simulink model "P702_NI_SoftECU"  (R2019a)
settings: Solver=ode1  StartTime=0.0  StopTime=Inf  FixedStep=0.001  RelTol=1e-3  EnableMultiTasking=on
PreLoadFcn:
  | run '.\VeriStand_BlockSet\NIVeriStandAddPaths.m'
undefined symbols (not defined in the file or in its folder): magnitude
libraries: simulink x83, simulink_extras x1
(part 63 of 76)

== system P702_NI_SoftECU/SoftECU/SCCM/Mapping/Steering_Data ==
  In1 : Inport
  Bus Selector : BusSelector  OutputSignals=AhbStat_B_Dsply,HeadLghtHiCtrl_D_RqAhb,HeadLghtHiOn_B_StatAhb,CcButtnOnPress,CcButtnOffPress,CcAslButtnCnclPress,CcAsllButtnResPress,CcAslButtnResIncPress,CcAslButtnSetIncPress,CcAslButtnSetDecPress,CcAslButtnSetPress,AccButtnGapIncPress,AccButtnGapDecPress,AslButtnOnOffPress,AslButtnOnOffCnclPress,CcButtnOnOffPress,CcButtnOnOffCnclPress,CcAslButtnResDecPress,CcAslButtnOnPress,CcAslButtnCnclResPress
  Gain{,1..19} (20 alike) : Gain
  buscreator : BusCreator  Inputs=20
  Out1 : Outport
  wires:
  buscreator/1 -> Out1/1  "Steering_Data"
  Bus Selector/1 -> Gain19/1  "<AhbStat_B_Dsply>"
  Bus Selector/2 -> Gain18/1  "<HeadLghtHiCtrl_D_RqAhb>"
  Bus Selector/3 -> Gain17/1  "<HeadLghtHiOn_B_StatAhb>"
  In1/1 -> Bus Selector/1
  Gain19/1 -> buscreator/1  "AhbStat_B_Dsply"
  Gain18/1 -> buscreator/2  "HeadLghtHiCtrl_D_RqAhb"
  Gain17/1 -> buscreator/3  "HeadLghtHiOn_B_StatAhb"
  Bus Selector/7 -> Gain13/1  "<CcAsllButtnResPress>"
  Bus Selector/5 -> Gain15/1  "<CcButtnOffPress>"
  Bus Selector/6 -> Gain14/1  "<CcAslButtnCnclPress>"
  Bus Selector/4 -> Gain16/1  "<CcButtnOnPress>"
  Bus Selector/8 -> Gain/1  "<CcAslButtnResIncPress>"
  Bus Selector/9 -> Gain1/1  "<CcAslButtnSetIncPress>"
  Bus Selector/10 -> Gain2/1  "<CcAslButtnSetDecPress>"
  Gain15/1 -> buscreator/5  "CcButtnOffPress"
  Gain1/1 -> buscreator/9  "CcAslButtnSetIncPress"
  Gain14/1 -> buscreator/6  "CcAslButtnCnclPress"
  Gain/1 -> buscreator/8  "CcAslButtnResIncPress"
  Gain13/1 -> buscreator/7  "CcAsllButtnResPress"
  Gain16/1 -> buscreator/4  "CcButtnOnPress"
  Gain2/1 -> buscreator/10  "CcAslButtnSetDecPress"
  Bus Selector/11 -> Gain3/1  "<CcAslButtnSetPress>"
  Gain3/1 -> buscreator/11  "CcAslButtnSetPress"
  Bus Selector/17 -> Gain9/1  "<CcButtnOnOffCnclPress>"
  Bus Selector/19 -> Gain11/1  "<CcAslButtnOnPress>"
  Bus Selector/15 -> Gain7/1  "<AslButtnOnOffCnclPress>"
  Bus Selector/16 -> Gain8/1  "<CcButtnOnOffPress>"
  Bus Selector/13 -> Gain5/1  "<AccButtnGapDecPress>"
  Bus Selector/20 -> Gain12/1  "<CcAslButtnCnclResPress>"
  Bus Selector/12 -> Gain4/1  "<AccButtnGapIncPress>"
  Bus Selector/14 -> Gain6/1  "<AslButtnOnOffPress>"
  Bus Selector/18 -> Gain10/1  "<CcAslButtnResDecPress>"
  Gain6/1 -> buscreator/14  "AslButtnOnOffPress"
  Gain7/1 -> buscreator/15  "AslButtnOnOffCnclPress"
  Gain5/1 -> buscreator/13  "AccButtnGapDecPress"
  Gain4/1 -> buscreator/12  "AccButtnGapIncPress"
  Gain11/1 -> buscreator/19  "CcAslButtnOnPress"
  Gain9/1 -> buscreator/17  "CcButtnOnOffCnclPress"
  Gain8/1 -> buscreator/16  "CcButtnOnOffPress"
  Gain12/1 -> buscreator/20  "CcAslButtnCnclResPress"
  Gain10/1 -> buscreator/18  "CcAslButtnResDecPress"

== system P702_NI_SoftECU/SoftECU/SCCM/Mapping/Steering_Wheel_Data2 ==
  In1 : Inport
  Bus Creator6 : BusCreator  Inputs=7
  Bus Selector : BusSelector  OutputSignals=SteWhlSwtchOk_B_Stat,SteeringWheelTglBtnUp_B,SteeringWheelTglBtnDown_B,SteeringWheelTglBtnLeft_B,SteeringWheelTglBtnRight_B,SteeringWheelTglBtnMenue_B,SteeringWheelTglBtnBack_B
  Gain{,1..6} (7 alike) : Gain
  Out1 : Outport
  wires:
  Bus Creator6/1 -> Out1/1  "Steering_Wheel_Data2"
  Gain/1 -> Bus Creator6/1  "SteWhlSwtchOk_B_Stat"
  Gain1/1 -> Bus Creator6/2  "SteWhlSwtchUp_B_Stat"
  Gain2/1 -> Bus Creator6/3  "SteWhlSwtchDown_B_Stat"
  Gain3/1 -> Bus Creator6/4  "SteWhlSwtchLeft_B_Stat"
  Gain4/1 -> Bus Creator6/5  "SteWhlSwtchRght_B_Stat"
  Gain5/1 -> Bus Creator6/6  "SteWhlSwtchMenu_B_Stat"
  In1/1 -> Bus Selector/1
  Bus Selector/2 -> Gain1/1  "<SteeringWheelTglBtnUp_B>"
  Bus Selector/3 -> Gain2/1  "<SteeringWheelTglBtnDown_B>"
  Bus Selector/1 -> Gain/1  "<SteWhlSwtchOk_B_Stat>"
  Bus Selector/4 -> Gain3/1  "<SteeringWheelTglBtnLeft_B>"
  Bus Selector/5 -> Gain4/1  "<SteeringWheelTglBtnRight_B>"
  Bus Selector/6 -> Gain5/1  "<SteeringWheelTglBtnMenue_B>"
  Bus Selector/7 -> Gain6/1  "<SteeringWheelTglBtnBack_B>"
  Gain6/1 -> Bus Creator6/7  "SteWhlSwtchBack_B_Stat"

== system P702_NI_SoftECU/SoftECU/SRR_L/FrontLeft_SOD/SRR_FL_001 ==
  target_pos : Inport
  sensor_pos : Inport  Port=2
  CSP : Inport  Port=3
  Bus Creator : BusCreator  Inputs=7
  Compare To Constant : simulink/Logic and Bit Operations/Compare To Constant  relop=~=  const=-1  OutDataTypeStr=boolean
  Data Type Conversion{,1..7} (8 alike) : DataTypeConversion
  Gain : Gain  Gain=24
  SUPER_RES_TARGET : Constant  Value=0
  Subsystem : Subsystem
  SRR_FL_001 : Outport
  wires:
  Data Type Conversion6/1 -> Bus Creator/7  "SRR_FL_CAN_DET_VALID_LEVEL_01"
  Data Type Conversion7/1 -> Bus Creator/6  "SRR_FL_CAN_DET_AMPLITUDE_01"
  Data Type Conversion5/1 -> Bus Creator/5  "SRR_FL_CAN_DET_SUPER_RES_TARGET_01"
  Data Type Conversion4/1 -> Bus Creator/4  "SRR_FL_CAN_DET_ELEVATION_01"
  Data Type Conversion3/1 -> Bus Creator/3  "SRR_FL_CAN_DET_AZIMUTH_01"
  Data Type Conversion2/1 -> Bus Creator/2  "SRR_FL_CAN_DET_RANGE_RATE_01"
  Data Type Conversion1/1 -> Bus Creator/1  "SRR_FL_CAN_DET_RANGE_01"
  Data Type Conversion/1 -> Gain/1
  Gain/1 -> Data Type Conversion7/1
  Compare To Constant/1 -> Data Type Conversion/1, Data Type Conversion6/1
  SUPER_RES_TARGET/1 -> Data Type Conversion5/1
  Subsystem/4(elevation) -> Data Type Conversion4/1
  Subsystem/3(azimuth) -> Data Type Conversion3/1
  Subsystem/2(range_rate) -> Data Type Conversion2/1
  Subsystem/1(range) -> Data Type Conversion1/1, Compare To Constant/1
  CSP/1 -> Subsystem/3(CSP)
  sensor_pos/1 -> Subsystem/2(sensor_pos)
  target_pos/1 -> Subsystem/1(target_pos)
  Bus Creator/1 -> SRR_FL_001/1

== system P702_NI_SoftECU/SoftECU/SRR_L/FrontLeft_SOD/SRR_FL_002 ==
  target_pos : Inport
  sensor_pos : Inport  Port=2
  CSP : Inport  Port=3
  Bus Creator : BusCreator  Inputs=7
  Compare To Constant : simulink/Logic and Bit Operations/Compare To Constant  relop=~=  const=-1  OutDataTypeStr=boolean
  Data Type Conversion{,1..7} (8 alike) : DataTypeConversion
  Gain : Gain  Gain=24
  SUPER_RES_TARGET : Constant  Value=0
  Subsystem : Subsystem
  SRR_FL_002 : Outport
  wires:
  target_pos/1 -> Subsystem/1(target_pos)
  sensor_pos/1 -> Subsystem/2(sensor_pos)
  CSP/1 -> Subsystem/3(CSP)
  Subsystem/1(range) -> Compare To Constant/1, Data Type Conversion1/1
  Subsystem/2(range_rate) -> Data Type Conversion2/1
  Subsystem/3(azimuth) -> Data Type Conversion3/1
  Subsystem/4(elevation) -> Data Type Conversion4/1
  SUPER_RES_TARGET/1 -> Data Type Conversion5/1
  Compare To Constant/1 -> Data Type Conversion6/1, Data Type Conversion/1
  Gain/1 -> Data Type Conversion7/1
  Data Type Conversion/1 -> Gain/1
  Data Type Conversion1/1 -> Bus Creator/1  "SRR_FL_CAN_DET_RANGE_02"
  Data Type Conversion2/1 -> Bus Creator/2  "SRR_FL_CAN_DET_RANGE_RATE_02"
  Data Type Conversion3/1 -> Bus Creator/3  "SRR_FL_CAN_DET_AZIMUTH_02"
  Data Type Conversion4/1 -> Bus Creator/4  "SRR_FL_CAN_DET_ELEVATION_02"
  Data Type Conversion5/1 -> Bus Creator/5  "SRR_FL_CAN_DET_SUPER_RES_TARGET_02"
  Data Type Conversion7/1 -> Bus Creator/6  "SRR_FL_CAN_DET_AMPLITUDE_02"
  Data Type Conversion6/1 -> Bus Creator/7  "SRR_FL_CAN_DET_VALID_LEVEL_02"
  Bus Creator/1 -> SRR_FL_002/1

== system P702_NI_SoftECU/SoftECU/SRR_L/FrontLeft_SOD/SRR_FL_003 ==
  target_pos : Inport
  sensor_pos : Inport  Port=2
  CSP : Inport  Port=3
  Bus Creator : BusCreator  Inputs=7
  Compare To Constant : simulink/Logic and Bit Operations/Compare To Constant  relop=~=  const=-1  OutDataTypeStr=boolean
  Data Type Conversion{,1..7} (8 alike) : DataTypeConversion
  Gain : Gain  Gain=24
  SUPER_RES_TARGET : Constant  Value=0
  Subsystem : Subsystem
  SRR_FL_003 : Outport
  wires:
  Data Type Conversion6/1 -> Bus Creator/7  "SRR_FL_CAN_DET_VALID_LEVEL_03"
  Data Type Conversion7/1 -> Bus Creator/6  "SRR_FL_CAN_DET_AMPLITUDE_03"
  Data Type Conversion5/1 -> Bus Creator/5  "SRR_FL_CAN_DET_SUPER_RES_TARGET_03"
  Data Type Conversion4/1 -> Bus Creator/4  "SRR_FL_CAN_DET_ELEVATION_03"
  Data Type Conversion3/1 -> Bus Creator/3  "SRR_FL_CAN_DET_AZIMUTH_03"
  Data Type Conversion2/1 -> Bus Creator/2  "SRR_FL_CAN_DET_RANGE_RATE_03"
  Data Type Conversion1/1 -> Bus Creator/1  "SRR_FL_CAN_DET_RANGE_03"
  Data Type Conversion/1 -> Gain/1
  Gain/1 -> Data Type Conversion7/1
  Compare To Constant/1 -> Data Type Conversion/1, Data Type Conversion6/1
  SUPER_RES_TARGET/1 -> Data Type Conversion5/1
  Subsystem/4(elevation) -> Data Type Conversion4/1
  Subsystem/3(azimuth) -> Data Type Conversion3/1
  Subsystem/2(range_rate) -> Data Type Conversion2/1
  Subsystem/1(range) -> Data Type Conversion1/1, Compare To Constant/1
  CSP/1 -> Subsystem/3(CSP)
  sensor_pos/1 -> Subsystem/2(sensor_pos)
  target_pos/1 -> Subsystem/1(target_pos)
  Bus Creator/1 -> SRR_FL_003/1

== system P702_NI_SoftECU/SoftECU/SRR_L/RearLeft_SOD/SRR_RL_001  ==
  target_pos : Inport
  sensor_pos : Inport  Port=2
  CSP : Inport  Port=3
  Bus Creator : BusCreator  Inputs=7
  Compare To Constant : simulink/Logic and Bit Operations/Compare To Constant  relop=~=  const=-1  OutDataTypeStr=boolean
  Data Type Conversion{,1..7} (8 alike) : DataTypeConversion
  Gain : Gain  Gain=24
  SRR_RL_CAN_DET_AZIMUTH_01 : S-Function  Priority=2  FunctionName=NIVeriStandIO  Parameters=width dtype portnum stime stype btype  SFunctionDeploymentMode=off  EnableBusSupport=off  mask(NI VeriStand Outport){portnum=2, width=-1, stime=-1, dtype=auto, stype=auto, btype=0}
      mask prompts: portnum "Port number:"; width "Port dimensions (-1 for dynamically sized):"; stime "Sample time (-1 for inherited):"; dtype "Data type:"; stype "Signal type:"; btype "Block type:"
      mask help: Use this outport on any level of nested subsystems to allow NI VeriStand software to map signals to it.
      mask init:
      | NIVeriStandIO_init;
      settings: CopyFcn=NIVeriStand_MDL_functions('', 'IO_copy');  DeleteFcn=NIVeriStand_MDL_functions('', 'IO_delete');  MoveFcn=set_param(gcb, 'Mask', 'on');
      mask Callback portnum: NIVeriStand_MDL_functions('', 'IO_setportnum');
      mask TypeOptions dtype: auto | double | single | int8 | uint8 | int16 | uint16 | int32 | uint32 | boolean
      mask Callback dtype: NIVeriStand_MDL_functions('', 'IO_booleansignal');
      mask TypeOptions stype: auto | real | complex
      mask Display:
      | patch([-x x], [-y y], [.90980 .81960 .32156]);
      | plot([xrad -x x xrad], [yrad -y y yrad]);
      | fprintf('NI Out%d', portnum);
  SRR_RL_CAN_DET_RANGE_01 : S-Function  Priority=1  FunctionName=NIVeriStandIO  Parameters=width dtype portnum stime stype btype  SFunctionDeploymentMode=off  EnableBusSupport=off  mask(NI VeriStand Outport){portnum=1, width=-1, stime=-1, dtype=auto, stype=auto, btype=0}
      mask prompts: portnum "Port number:"; width "Port dimensions (-1 for dynamically sized):"; stime "Sample time (-1 for inherited):"; dtype "Data type:"; stype "Signal type:"; btype "Block type:"
      mask help: Use this outport on any level of nested subsystems to allow NI VeriStand software to map signals to it.
      mask init:
      | NIVeriStandIO_init;
      settings: CopyFcn=NIVeriStand_MDL_functions('', 'IO_copy');  DeleteFcn=NIVeriStand_MDL_functions('', 'IO_delete');  MoveFcn=set_param(gcb, 'Mask', 'on');
      mask Callback portnum: NIVeriStand_MDL_functions('', 'IO_setportnum');
      mask TypeOptions dtype: auto | double | single | int8 | uint8 | int16 | uint16 | int32 | uint32 | boolean
      mask Callback dtype: NIVeriStand_MDL_functions('', 'IO_booleansignal');
      mask TypeOptions stype: auto | real | complex
      mask Display:
      | patch([-x x], [-y y], [.90980 .81960 .32156]);
      | plot([xrad -x x xrad], [yrad -y y yrad]);
      | fprintf('NI Out%d', portnum);
  SUPER_RES_TARGET : Constant  Value=0
  Subsystem : Subsystem
  SRR_RL_001 : Outport
  wires:
  target_pos/1 -> Subsystem/1(target_pos)
  sensor_pos/1 -> Subsystem/2(sensor_pos)
  CSP/1 -> Subsystem/3(CSP)
  Subsystem/1(range) -> Compare To Constant/1, Data Type Conversion1/1
  Subsystem/2(range_rate) -> Data Type Conversion2/1
  Subsystem/3(azimuth) -> Data Type Conversion3/1
  Subsystem/4(elevation) -> Data Type Conversion4/1
  SUPER_RES_TARGET/1 -> Data Type Conversion5/1
  Compare To Constant/1 -> Data Type Conversion6/1, Data Type Conversion/1
  Gain/1 -> Data Type Conversion7/1
  Data Type Conversion/1 -> Gain/1
  Data Type Conversion1/1 -> SRR_RL_CAN_DET_RANGE_01/1, Bus Creator/1  "SRR_RL_CAN_DET_RANGE_01"
  Data Type Conversion2/1 -> Bus Creator/2  "SRR_RL_CAN_DET_RANGE_RATE_01"
  Data Type Conversion3/1 -> SRR_RL_CAN_DET_AZIMUTH_01/1, Bus Creator/3  "SRR_RL_CAN_DET_AZIMUTH_01"
  Data Type Conversion4/1 -> Bus Creator/4  "SRR_RL_CAN_DET_ELEVATION_01"
  Data Type Conversion5/1 -> Bus Creator/5  "SRR_RL_CAN_DET_SUPER_RES_TARGET_01"
  Data Type Conversion7/1 -> Bus Creator/6  "SRR_RL_CAN_DET_AMPLITUDE_01"
  Data Type Conversion6/1 -> Bus Creator/7  "SRR_RL_CAN_DET_VALID_LEVEL_01"
  Bus Creator/1 -> SRR_RL_001/1

== system P702_NI_SoftECU/SoftECU/SRR_L/RearLeft_SOD/SRR_RL_002 ==
  target_pos : Inport
  sensor_pos : Inport  Port=2
  CSP : Inport  Port=3
  Bus Creator : BusCreator  Inputs=7
  Compare To Constant : simulink/Logic and Bit Operations/Compare To Constant  relop=~=  const=-1  OutDataTypeStr=boolean
  Data Type Conversion{,1..7} (8 alike) : DataTypeConversion
  Gain : Gain  Gain=24
  SRR_RL_CAN_DET_AZIMUTH_02 : S-Function  Priority=2  FunctionName=NIVeriStandIO  Parameters=width dtype portnum stime stype btype  SFunctionDeploymentMode=off  EnableBusSupport=off  mask(NI VeriStand Outport){portnum=2, width=-1, stime=-1, dtype=auto, stype=auto, btype=0}
      mask prompts: portnum "Port number:"; width "Port dimensions (-1 for dynamically sized):"; stime "Sample time (-1 for inherited):"; dtype "Data type:"; stype "Signal type:"; btype "Block type:"
      mask help: Use this outport on any level of nested subsystems to allow NI VeriStand software to map signals to it.
      mask init:
      | NIVeriStandIO_init;
      settings: CopyFcn=NIVeriStand_MDL_functions('', 'IO_copy');  DeleteFcn=NIVeriStand_MDL_functions('', 'IO_delete');  MoveFcn=set_param(gcb, 'Mask', 'on');
      mask Callback portnum: NIVeriStand_MDL_functions('', 'IO_setportnum');
      mask TypeOptions dtype: auto | double | single | int8 | uint8 | int16 | uint16 | int32 | uint32 | boolean
      mask Callback dtype: NIVeriStand_MDL_functions('', 'IO_booleansignal');
      mask TypeOptions stype: auto | real | complex
      mask Display:
      | patch([-x x], [-y y], [.90980 .81960 .32156]);
      | plot([xrad -x x xrad], [yrad -y y yrad]);
      | fprintf('NI Out%d', portnum);
  SRR_RL_CAN_DET_RANGE_02 : S-Function  Priority=1  FunctionName=NIVeriStandIO  Parameters=width dtype portnum stime stype btype  SFunctionDeploymentMode=off  EnableBusSupport=off  mask(NI VeriStand Outport){portnum=1, width=-1, stime=-1, dtype=auto, stype=auto, btype=0}
      mask prompts: portnum "Port number:"; width "Port dimensions (-1 for dynamically sized):"; stime "Sample time (-1 for inherited):"; dtype "Data type:"; stype "Signal type:"; btype "Block type:"
      mask help: Use this outport on any level of nested subsystems to allow NI VeriStand software to map signals to it.
      mask init:
      | NIVeriStandIO_init;
      settings: CopyFcn=NIVeriStand_MDL_functions('', 'IO_copy');  DeleteFcn=NIVeriStand_MDL_functions('', 'IO_delete');  MoveFcn=set_param(gcb, 'Mask', 'on');
      mask Callback portnum: NIVeriStand_MDL_functions('', 'IO_setportnum');
      mask TypeOptions dtype: auto | double | single | int8 | uint8 | int16 | uint16 | int32 | uint32 | boolean
      mask Callback dtype: NIVeriStand_MDL_functions('', 'IO_booleansignal');
      mask TypeOptions stype: auto | real | complex
      mask Display:
      | patch([-x x], [-y y], [.90980 .81960 .32156]);
      | plot([xrad -x x xrad], [yrad -y y yrad]);
      | fprintf('NI Out%d', portnum);
  SUPER_RES_TARGET : Constant  Value=0
  Subsystem : Subsystem
  SRR_RL_002 : Outport
  wires:
  Data Type Conversion6/1 -> Bus Creator/7  "SRR_RL_CAN_DET_VALID_LEVEL_02"
  Data Type Conversion7/1 -> Bus Creator/6  "SRR_RL_CAN_DET_AMPLITUDE_02"
  Data Type Conversion5/1 -> Bus Creator/5  "SRR_RL_CAN_DET_SUPER_RES_TARGET_02"
  Data Type Conversion4/1 -> Bus Creator/4  "SRR_RL_CAN_DET_ELEVATION_02"
  Data Type Conversion3/1 -> SRR_RL_CAN_DET_AZIMUTH_02/1, Bus Creator/3  "SRR_RL_CAN_DET_AZIMUTH_02"
  Data Type Conversion2/1 -> Bus Creator/2  "SRR_RL_CAN_DET_RANGE_RATE_02"
  Data Type Conversion1/1 -> SRR_RL_CAN_DET_RANGE_02/1, Bus Creator/1  "SRR_RL_CAN_DET_RANGE_02"
  Data Type Conversion/1 -> Gain/1
  Gain/1 -> Data Type Conversion7/1
  Compare To Constant/1 -> Data Type Conversion/1, Data Type Conversion6/1
  SUPER_RES_TARGET/1 -> Data Type Conversion5/1
  Subsystem/4(elevation) -> Data Type Conversion4/1
  Subsystem/3(azimuth) -> Data Type Conversion3/1
  Subsystem/2(range_rate) -> Data Type Conversion2/1
  Subsystem/1(range) -> Data Type Conversion1/1, Compare To Constant/1
  CSP/1 -> Subsystem/3(CSP)
  sensor_pos/1 -> Subsystem/2(sensor_pos)
  target_pos/1 -> Subsystem/1(target_pos)
  Bus Creator/1 -> SRR_RL_002/1

== system P702_NI_SoftECU/SoftECU/SRR_L/RearLeft_SOD/SRR_RL_003 ==
  target_pos : Inport
  sensor_pos : Inport  Port=2
  CSP : Inport  Port=3
  Bus Creator : BusCreator  Inputs=7
  Compare To Constant : simulink/Logic and Bit Operations/Compare To Constant  relop=~=  const=-1  OutDataTypeStr=boolean
  Data Type Conversion{,1..7} (8 alike) : DataTypeConversion
  Gain : Gain  Gain=24
  SRR_RL_CAN_DET_AZIMUTH_03 : S-Function  Priority=2  FunctionName=NIVeriStandIO  Parameters=width dtype portnum stime stype btype  SFunctionDeploymentMode=off  EnableBusSupport=off  mask(NI VeriStand Outport){portnum=2, width=-1, stime=-1, dtype=auto, stype=auto, btype=0}
      mask prompts: portnum "Port number:"; width "Port dimensions (-1 for dynamically sized):"; stime "Sample time (-1 for inherited):"; dtype "Data type:"; stype "Signal type:"; btype "Block type:"
      mask help: Use this outport on any level of nested subsystems to allow NI VeriStand software to map signals to it.
      mask init:
      | NIVeriStandIO_init;
      settings: CopyFcn=NIVeriStand_MDL_functions('', 'IO_copy');  DeleteFcn=NIVeriStand_MDL_functions('', 'IO_delete');  MoveFcn=set_param(gcb, 'Mask', 'on');
      mask Callback portnum: NIVeriStand_MDL_functions('', 'IO_setportnum');
      mask TypeOptions dtype: auto | double | single | int8 | uint8 | int16 | uint16 | int32 | uint32 | boolean
      mask Callback dtype: NIVeriStand_MDL_functions('', 'IO_booleansignal');
      mask TypeOptions stype: auto | real | complex
      mask Display:
      | patch([-x x], [-y y], [.90980 .81960 .32156]);
      | plot([xrad -x x xrad], [yrad -y y yrad]);
      | fprintf('NI Out%d', portnum);
  SRR_RL_CAN_DET_RANGE_03 : S-Function  Priority=1  FunctionName=NIVeriStandIO  Parameters=width dtype portnum stime stype btype  SFunctionDeploymentMode=off  EnableBusSupport=off  mask(NI VeriStand Outport){portnum=1, width=-1, stime=-1, dtype=auto, stype=auto, btype=0}
      mask prompts: portnum "Port number:"; width "Port dimensions (-1 for dynamically sized):"; stime "Sample time (-1 for inherited):"; dtype "Data type:"; stype "Signal type:"; btype "Block type:"
      mask help: Use this outport on any level of nested subsystems to allow NI VeriStand software to map signals to it.
      mask init:
      | NIVeriStandIO_init;
      settings: CopyFcn=NIVeriStand_MDL_functions('', 'IO_copy');  DeleteFcn=NIVeriStand_MDL_functions('', 'IO_delete');  MoveFcn=set_param(gcb, 'Mask', 'on');
      mask Callback portnum: NIVeriStand_MDL_functions('', 'IO_setportnum');
      mask TypeOptions dtype: auto | double | single | int8 | uint8 | int16 | uint16 | int32 | uint32 | boolean
      mask Callback dtype: NIVeriStand_MDL_functions('', 'IO_booleansignal');
      mask TypeOptions stype: auto | real | complex
      mask Display:
      | patch([-x x], [-y y], [.90980 .81960 .32156]);
      | plot([xrad -x x xrad], [yrad -y y yrad]);
      | fprintf('NI Out%d', portnum);
  SUPER_RES_TARGET : Constant  Value=0
  Subsystem : Subsystem
  SRR_RL_003 : Outport
  wires:
  target_pos/1 -> Subsystem/1(target_pos)
  sensor_pos/1 -> Subsystem/2(sensor_pos)
  CSP/1 -> Subsystem/3(CSP)
  Subsystem/1(range) -> Compare To Constant/1, Data Type Conversion1/1
  Subsystem/2(range_rate) -> Data Type Conversion2/1
  Subsystem/3(azimuth) -> Data Type Conversion3/1
  Subsystem/4(elevation) -> Data Type Conversion4/1
  SUPER_RES_TARGET/1 -> Data Type Conversion5/1
  Compare To Constant/1 -> Data Type Conversion6/1, Data Type Conversion/1
  Gain/1 -> Data Type Conversion7/1
  Data Type Conversion/1 -> Gain/1
  Data Type Conversion1/1 -> SRR_RL_CAN_DET_RANGE_03/1, Bus Creator/1  "SRR_RL_CAN_DET_RANGE_03"
  Data Type Conversion2/1 -> Bus Creator/2  "SRR_RL_CAN_DET_RANGE_RATE_03"
  Data Type Conversion3/1 -> SRR_RL_CAN_DET_AZIMUTH_03/1, Bus Creator/3  "SRR_RL_CAN_DET_AZIMUTH_03"
  Data Type Conversion4/1 -> Bus Creator/4  "SRR_RL_CAN_DET_ELEVATION_03"
  Data Type Conversion5/1 -> Bus Creator/5  "SRR_RL_CAN_DET_SUPER_RES_TARGET_03"
  Data Type Conversion7/1 -> Bus Creator/6  "SRR_RL_CAN_DET_AMPLITUDE_03"
  Data Type Conversion6/1 -> Bus Creator/7  "SRR_RL_CAN_DET_VALID_LEVEL_03"
  Bus Creator/1 -> SRR_RL_003/1

== system P702_NI_SoftECU/SoftECU/SRR_R/FrontRight_SOD/SRR_FR_001  ==
  target_pos : Inport
  sensor_pos : Inport  Port=2
  CSP : Inport  Port=3
  Bus Creator : BusCreator  Inputs=7
  Compare To Constant : simulink/Logic and Bit Operations/Compare To Constant  relop=~=  const=-1  OutDataTypeStr=boolean
  Data Type Conversion{,1..7} (8 alike) : DataTypeConversion
  Gain : Gain  Gain=24
  SUPER_RES_TARGET : Constant  Value=0
  Subsystem : Subsystem
  SRR_FR_001 : Outport
  wires:
  Data Type Conversion6/1 -> Bus Creator/7  "SRR_FR_CAN_DET_VALID_LEVEL_01"
  Data Type Conversion7/1 -> Bus Creator/6  "SRR_FR_CAN_DET_AMPLITUDE_01"
  Data Type Conversion5/1 -> Bus Creator/5  "SRR_FR_CAN_DET_SUPER_RES_TARGET_01"
  Data Type Conversion4/1 -> Bus Creator/4  "SRR_FR_CAN_DET_ELEVATION_01"
  Data Type Conversion3/1 -> Bus Creator/3  "SRR_FR_CAN_DET_AZIMUTH_01"
  Data Type Conversion2/1 -> Bus Creator/2  "SRR_FR_CAN_DET_RANGE_RATE_01"
  Data Type Conversion1/1 -> Bus Creator/1  "SRR_FR_CAN_DET_RANGE_01"
  Data Type Conversion/1 -> Gain/1
  Gain/1 -> Data Type Conversion7/1
  Compare To Constant/1 -> Data Type Conversion/1, Data Type Conversion6/1
  SUPER_RES_TARGET/1 -> Data Type Conversion5/1
  Subsystem/4(elevation) -> Data Type Conversion4/1
  Subsystem/3(azimuth) -> Data Type Conversion3/1
  Subsystem/2(range_rate) -> Data Type Conversion2/1
  Subsystem/1(range) -> Data Type Conversion1/1, Compare To Constant/1
  CSP/1 -> Subsystem/3(CSP)
  sensor_pos/1 -> Subsystem/2(sensor_pos)
  target_pos/1 -> Subsystem/1(target_pos)
  Bus Creator/1 -> SRR_FR_001/1

== system P702_NI_SoftECU/SoftECU/SRR_R/FrontRight_SOD/SRR_FR_002 ==
  target_pos : Inport
  sensor_pos : Inport  Port=2
  CSP : Inport  Port=3
  Bus Creator : BusCreator  Inputs=7
  Compare To Constant : simulink/Logic and Bit Operations/Compare To Constant  relop=~=  const=-1  OutDataTypeStr=boolean
  Data Type Conversion{,1..7} (8 alike) : DataTypeConversion
  Gain : Gain  Gain=24
  SUPER_RES_TARGET : Constant  Value=0
  Subsystem : Subsystem
  SRR_FR_002 : Outport
  wires:
  target_pos/1 -> Subsystem/1(target_pos)
  sensor_pos/1 -> Subsystem/2(sensor_pos)
  CSP/1 -> Subsystem/3(CSP)
  Subsystem/1(range) -> Compare To Constant/1, Data Type Conversion1/1
  Subsystem/2(range_rate) -> Data Type Conversion2/1
  Subsystem/3(azimuth) -> Data Type Conversion3/1
  Subsystem/4(elevation) -> Data Type Conversion4/1
  SUPER_RES_TARGET/1 -> Data Type Conversion5/1
  Compare To Constant/1 -> Data Type Conversion6/1, Data Type Conversion/1
  Gain/1 -> Data Type Conversion7/1
  Data Type Conversion/1 -> Gain/1
  Data Type Conversion1/1 -> Bus Creator/1  "SRR_FR_CAN_DET_RANGE_02"
  Data Type Conversion2/1 -> Bus Creator/2  "SRR_FR_CAN_DET_RANGE_RATE_02"
  Data Type Conversion3/1 -> Bus Creator/3  "SRR_FR_CAN_DET_AZIMUTH_02"
  Data Type Conversion4/1 -> Bus Creator/4  "SRR_FR_CAN_DET_ELEVATION_02"
  Data Type Conversion5/1 -> Bus Creator/5  "SRR_FR_CAN_DET_SUPER_RES_TARGET_02"
  Data Type Conversion7/1 -> Bus Creator/6  "SRR_FR_CAN_DET_AMPLITUDE_02"
  Data Type Conversion6/1 -> Bus Creator/7  "SRR_FR_CAN_DET_VALID_LEVEL_02"
  Bus Creator/1 -> SRR_FR_002/1

== system P702_NI_SoftECU/SoftECU/SRR_R/FrontRight_SOD/SRR_FR_003 ==
  target_pos : Inport
  sensor_pos : Inport  Port=2
  CSP : Inport  Port=3
  Bus Creator : BusCreator  Inputs=7
  Compare To Constant : simulink/Logic and Bit Operations/Compare To Constant  relop=~=  const=-1  OutDataTypeStr=boolean
  Data Type Conversion{,1..7} (8 alike) : DataTypeConversion
  Gain : Gain  Gain=24
  SUPER_RES_TARGET : Constant  Value=0
  Subsystem : Subsystem
  SRR_FR_003 : Outport
  wires:
  Data Type Conversion6/1 -> Bus Creator/7  "SRR_FR_CAN_DET_VALID_LEVEL_03"
  Data Type Conversion7/1 -> Bus Creator/6  "SRR_FR_CAN_DET_AMPLITUDE_03"
  Data Type Conversion5/1 -> Bus Creator/5  "SRR_FR_CAN_DET_SUPER_RES_TARGET_03"
  Data Type Conversion4/1 -> Bus Creator/4  "SRR_FR_CAN_DET_ELEVATION_03"
  Data Type Conversion3/1 -> Bus Creator/3  "SRR_FR_CAN_DET_AZIMUTH_03"
  Data Type Conversion2/1 -> Bus Creator/2  "SRR_FR_CAN_DET_RANGE_RATE_03"
  Data Type Conversion1/1 -> Bus Creator/1  "SRR_FR_CAN_DET_RANGE_03"
  Data Type Conversion/1 -> Gain/1
  Gain/1 -> Data Type Conversion7/1
  Compare To Constant/1 -> Data Type Conversion/1, Data Type Conversion6/1
  SUPER_RES_TARGET/1 -> Data Type Conversion5/1
  Subsystem/4(elevation) -> Data Type Conversion4/1
  Subsystem/3(azimuth) -> Data Type Conversion3/1
  Subsystem/2(range_rate) -> Data Type Conversion2/1
  Subsystem/1(range) -> Data Type Conversion1/1, Compare To Constant/1
  CSP/1 -> Subsystem/3(CSP)
  sensor_pos/1 -> Subsystem/2(sensor_pos)
  target_pos/1 -> Subsystem/1(target_pos)
  Bus Creator/1 -> SRR_FR_003/1

== system P702_NI_SoftECU/SoftECU/SRR_R/RearRight_SOD/SRR_RR_001  ==
  target_pos : Inport
  sensor_pos : Inport  Port=2
  CSP : Inport  Port=3
  Bus Creator : BusCreator  Inputs=7
  Compare To Constant : simulink/Logic and Bit Operations/Compare To Constant  relop=~=  const=-1  OutDataTypeStr=boolean
  Data Type Conversion{,1..7} (8 alike) : DataTypeConversion
  Gain : Gain  Gain=24
  SUPER_RES_TARGET : Constant  Value=0
  Subsystem : Subsystem
  SRR_RR_001 : Outport
  wires:
  target_pos/1 -> Subsystem/1(target_pos)
  sensor_pos/1 -> Subsystem/2(sensor_pos)
  CSP/1 -> Subsystem/3(CSP)
  Subsystem/1(range) -> Compare To Constant/1, Data Type Conversion1/1
  Subsystem/2(range_rate) -> Data Type Conversion2/1
  Subsystem/3(azimuth) -> Data Type Conversion3/1
  Subsystem/4(elevation) -> Data Type Conversion4/1
  SUPER_RES_TARGET/1 -> Data Type Conversion5/1
  Compare To Constant/1 -> Data Type Conversion6/1, Data Type Conversion/1
  Gain/1 -> Data Type Conversion7/1
  Data Type Conversion/1 -> Gain/1
  Data Type Conversion1/1 -> Bus Creator/1  "SRR_RR_CAN_DET_RANGE_01"
  Data Type Conversion2/1 -> Bus Creator/2  "SRR_RR_CAN_DET_RANGE_RATE_01"
  Data Type Conversion3/1 -> Bus Creator/3  "SRR_RR_CAN_DET_AZIMUTH_01"
  Data Type Conversion4/1 -> Bus Creator/4  "SRR_RR_CAN_DET_ELEVATION_01"
  Data Type Conversion5/1 -> Bus Creator/5  "SRR_RR_CAN_DET_SUPER_RES_TARGET_01"
  Data Type Conversion7/1 -> Bus Creator/6  "SRR_RR_CAN_DET_AMPLITUDE_01"
  Data Type Conversion6/1 -> Bus Creator/7  "SRR_RR_CAN_DET_VALID_LEVEL_01"
  Bus Creator/1 -> SRR_RR_001/1

== system P702_NI_SoftECU/SoftECU/SRR_R/RearRight_SOD/SRR_RR_002 ==
  target_pos : Inport
  sensor_pos : Inport  Port=2
  CSP : Inport  Port=3
  Bus Creator : BusCreator  Inputs=7
  Compare To Constant : simulink/Logic and Bit Operations/Compare To Constant  relop=~=  const=-1  OutDataTypeStr=boolean
  Data Type Conversion{,1..7} (8 alike) : DataTypeConversion
  Gain : Gain  Gain=24
  SUPER_RES_TARGET : Constant  Value=0
  Subsystem : Subsystem
  SRR_RR_002 : Outport
  wires:
  Data Type Conversion6/1 -> Bus Creator/7  "SRR_RR_CAN_DET_VALID_LEVEL_02"
  Data Type Conversion7/1 -> Bus Creator/6  "SRR_RR_CAN_DET_AMPLITUDE_02"
  Data Type Conversion5/1 -> Bus Creator/5  "SRR_RR_CAN_DET_SUPER_RES_TARGET_02"
  Data Type Conversion4/1 -> Bus Creator/4  "SRR_RR_CAN_DET_ELEVATION_02"
  Data Type Conversion3/1 -> Bus Creator/3  "SRR_RR_CAN_DET_AZIMUTH_02"
  Data Type Conversion2/1 -> Bus Creator/2  "SRR_RR_CAN_DET_RANGE_RATE_02"
  Data Type Conversion1/1 -> Bus Creator/1  "SRR_RR_CAN_DET_RANGE_02"
  Data Type Conversion/1 -> Gain/1
  Gain/1 -> Data Type Conversion7/1
  Compare To Constant/1 -> Data Type Conversion/1, Data Type Conversion6/1
  SUPER_RES_TARGET/1 -> Data Type Conversion5/1
  Subsystem/4(elevation) -> Data Type Conversion4/1
  Subsystem/3(azimuth) -> Data Type Conversion3/1
  Subsystem/2(range_rate) -> Data Type Conversion2/1
  Subsystem/1(range) -> Data Type Conversion1/1, Compare To Constant/1
  CSP/1 -> Subsystem/3(CSP)
  sensor_pos/1 -> Subsystem/2(sensor_pos)
  target_pos/1 -> Subsystem/1(target_pos)
  Bus Creator/1 -> SRR_RR_002/1

== system P702_NI_SoftECU/SoftECU/SRR_R/RearRight_SOD/SRR_RR_003 ==
  target_pos : Inport
  sensor_pos : Inport  Port=2
  CSP : Inport  Port=3
  Bus Creator : BusCreator  Inputs=7
  Compare To Constant : simulink/Logic and Bit Operations/Compare To Constant  relop=~=  const=-1  OutDataTypeStr=boolean
  Data Type Conversion{,1..7} (8 alike) : DataTypeConversion
  Gain : Gain  Gain=24
  SUPER_RES_TARGET : Constant  Value=0
  Subsystem : Subsystem
  SRR_RR_003 : Outport
  wires:
  target_pos/1 -> Subsystem/1(target_pos)
  sensor_pos/1 -> Subsystem/2(sensor_pos)
  CSP/1 -> Subsystem/3(CSP)
  Subsystem/1(range) -> Compare To Constant/1, Data Type Conversion1/1
  Subsystem/2(range_rate) -> Data Type Conversion2/1
  Subsystem/3(azimuth) -> Data Type Conversion3/1
  Subsystem/4(elevation) -> Data Type Conversion4/1
  SUPER_RES_TARGET/1 -> Data Type Conversion5/1
  Compare To Constant/1 -> Data Type Conversion6/1, Data Type Conversion/1
  Gain/1 -> Data Type Conversion7/1
  Data Type Conversion/1 -> Gain/1
  Data Type Conversion1/1 -> Bus Creator/1  "SRR_RR_CAN_DET_RANGE_03"
  Data Type Conversion2/1 -> Bus Creator/2  "SRR_RR_CAN_DET_RANGE_RATE_03"
  Data Type Conversion3/1 -> Bus Creator/3  "SRR_RR_CAN_DET_AZIMUTH_03"
  Data Type Conversion4/1 -> Bus Creator/4  "SRR_RR_CAN_DET_ELEVATION_03"
  Data Type Conversion5/1 -> Bus Creator/5  "SRR_RR_CAN_DET_SUPER_RES_TARGET_03"
  Data Type Conversion7/1 -> Bus Creator/6  "SRR_RR_CAN_DET_AMPLITUDE_03"
  Data Type Conversion6/1 -> Bus Creator/7  "SRR_RR_CAN_DET_VALID_LEVEL_03"
  Bus Creator/1 -> SRR_RR_003/1

== system P702_NI_SoftECU/SoftECU/TCM/Logic/ReValueStates ==
  note: SelectorLever[-3T|-2P|-1R|0N|1D]
  note: GearlvrPosDActl[-1Unknown|0P|1R|2N|3D]
  GearLvr[-] : Inport
  AddOffset_for_R-N_gears : Sum
  OffsetForSw : Constant  Value=2
  Transmission_Ratio[-] : Outport
  wires:
  AddOffset_for_R-N_gears/1 -> Transmission_Ratio[-]/1  "GearLvrPos_D_ActlPart"
  OffsetForSw/1 -> AddOffset_for_R-N_gears/2
  GearLvr[-]/1 -> AddOffset_for_R-N_gears/1

== system P702_NI_SoftECU/SoftECU/TCM/Mapping/TransGearData ==
  In1 : Inport
  Gain : Gain
  buscreator : BusCreator  Inputs=1
  busselector : BusSelector  OutputSignals=GearLvrPos_D_ActlPart
  Out1 : Outport
  wires:
  In1/1 -> busselector/1
  buscreator/1 -> Out1/1  "TransGearData"
  Gain/1 -> buscreator/1  "GearLvrPos_D_Actl"
  busselector/1 -> Gain/1  "<GearLvrPos_D_ActlPart>"

== system P702_NI_SoftECU/Output/Subsystem1/CAN_Signal/ABS_ESC/ABS_AutoSar_NetworkMgt_0x596 ==
  in_port : Inport
  ABS_AutoSarNMControl : Terminator
  ABS_AutoSarNMNodeId : Terminator
  ABS_AutoSarNMReserved{1..4} (4 alike) : Terminator
  ABS_GWNMProxy : Terminator
  ABS_GWOnBoardTester : Terminator
  bus_selector : BusSelector  OutputSignals=ABS_AutoSarNMNodeId,ABS_AutoSarNMControl,ABS_AutoSarNMReserved1,ABS_AutoSarNMReserved2,ABS_GWOnBoardTester,ABS_GWNMProxy,ABS_AutoSarNMReserved3,ABS_AutoSarNMReserved4
  wires:
  in_port/1 -> bus_selector/1  "Subsystem1"
  bus_selector/1 -> ABS_AutoSarNMNodeId/1  "<ABS_AutoSarNMNodeId>"
  bus_selector/2 -> ABS_AutoSarNMControl/1  "<ABS_AutoSarNMControl>"
  bus_selector/3 -> ABS_AutoSarNMReserved1/1  "<ABS_AutoSarNMReserved1>"
  bus_selector/4 -> ABS_AutoSarNMReserved2/1  "<ABS_AutoSarNMReserved2>"
  bus_selector/5 -> ABS_GWOnBoardTester/1  "<ABS_GWOnBoardTester>"
  bus_selector/6 -> ABS_GWNMProxy/1  "<ABS_GWNMProxy>"
  bus_selector/7 -> ABS_AutoSarNMReserved3/1  "<ABS_AutoSarNMReserved3>"
  bus_selector/8 -> ABS_AutoSarNMReserved4/1  "<ABS_AutoSarNMReserved4>"

== system P702_NI_SoftECU/Output/Subsystem1/CAN_Signal/ABS_ESC/ABS_BrkBst_Data_0x4B0 ==
  in_port : Inport
  BrkAutoHold_D_Stat : Terminator
  BrkBstrVac_P_Actl : Terminator
  BrkTotTqRqDrv_No_Cnt : Terminator
  BrkTotTqRqDrv_No_Cs : Terminator
  BrkTot_Tq_RqDrv : Terminator
  HsaStat_D_Dsply : Terminator
  HsaTrnAout_Tq_Rq : Terminator
  YawStabilityIndex : Terminator
  bus_selector : BusSelector  OutputSignals=BrkBstrVac_P_Actl,YawStabilityIndex,HsaTrnAout_Tq_Rq,BrkTotTqRqDrv_No_Cnt,BrkAutoHold_D_Stat,BrkTot_Tq_RqDrv,HsaStat_D_Dsply,BrkTotTqRqDrv_No_Cs
  wires:
  in_port/1 -> bus_selector/1  "Subsystem1"
  bus_selector/1 -> BrkBstrVac_P_Actl/1  "<BrkBstrVac_P_Actl>"
  bus_selector/2 -> YawStabilityIndex/1  "<YawStabilityIndex>"
  bus_selector/3 -> HsaTrnAout_Tq_Rq/1  "<HsaTrnAout_Tq_Rq>"
  bus_selector/4 -> BrkTotTqRqDrv_No_Cnt/1  "<BrkTotTqRqDrv_No_Cnt>"
  bus_selector/5 -> BrkAutoHold_D_Stat/1  "<BrkAutoHold_D_Stat>"
  bus_selector/6 -> BrkTot_Tq_RqDrv/1  "<BrkTot_Tq_RqDrv>"
  bus_selector/7 -> HsaStat_D_Dsply/1  "<HsaStat_D_Dsply>"
  bus_selector/8 -> BrkTotTqRqDrv_No_Cs/1  "<BrkTotTqRqDrv_No_Cs>"

== system P702_NI_SoftECU/Output/Subsystem1/CAN_Signal/ABS_ESC/ABS_Rapid_Data_Response_1_0x6B0 ==
  in_port : Inport
  UUDTABSResponse1 : Terminator
  bus_selector : BusSelector  OutputSignals=UUDTABSResponse1
  wires:
  in_port/1 -> bus_selector/1  "Subsystem1"
  bus_selector/1 -> UUDTABSResponse1/1  "<UUDTABSResponse1>"

== system P702_NI_SoftECU/Output/Subsystem1/CAN_Signal/ABS_ESC/ABS_Rapid_Data_Response_2_0x6B1 ==
  in_port : Inport
  UUDTABSResponse2 : Terminator
  bus_selector : BusSelector  OutputSignals=UUDTABSResponse2
  wires:
  in_port/1 -> bus_selector/1  "Subsystem1"
  bus_selector/1 -> UUDTABSResponse2/1  "<UUDTABSResponse2>"

== system P702_NI_SoftECU/Output/Subsystem1/CAN_Signal/ABS_ESC/ActiveFronSteering_Req_0x88 ==
  in_port : Inport
  SteWhlBrkAnRq_No_Cnt : Terminator
  SteWhlBrkAnRq_No_Cs : Terminator
  SteWhlBrkOffst_An_Rq : Terminator
  bus_selector : BusSelector  OutputSignals=SteWhlBrkOffst_An_Rq,SteWhlBrkAnRq_No_Cs,SteWhlBrkAnRq_No_Cnt
  wires:
  in_port/1 -> bus_selector/1  "Subsystem1"
  bus_selector/1 -> SteWhlBrkOffst_An_Rq/1  "<SteWhlBrkOffst_An_Rq>"
  bus_selector/2 -> SteWhlBrkAnRq_No_Cs/1  "<SteWhlBrkAnRq_No_Cs>"
  bus_selector/3 -> SteWhlBrkAnRq_No_Cnt/1  "<SteWhlBrkAnRq_No_Cnt>"

== system P702_NI_SoftECU/Output/Subsystem1/CAN_Signal/ABS_ESC/BrakeSnData_3_0x77 ==
  in_port : Inport
  VehLatComp_A_Actl : Terminator
  VehLongComp_A_Actl : Terminator
  VehOverGnd_V_Est : Terminator
  VehTrvlDir_D_Stat : Terminator
  VehYawComp_W_Actl : Terminator
  bus_selector : BusSelector  OutputSignals=VehOverGnd_V_Est,VehTrvlDir_D_Stat,VehYawComp_W_Actl,VehLatComp_A_Actl,VehLongComp_A_Actl
  wires:
  in_port/1 -> bus_selector/1  "Subsystem1"
  bus_selector/1 -> VehOverGnd_V_Est/1  "<VehOverGnd_V_Est>"
  bus_selector/2 -> VehTrvlDir_D_Stat/1  "<VehTrvlDir_D_Stat>"
  bus_selector/3 -> VehYawComp_W_Actl/1  "<VehYawComp_W_Actl>"
  bus_selector/4 -> VehLatComp_A_Actl/1  "<VehLatComp_A_Actl>"
  bus_selector/5 -> VehLongComp_A_Actl/1  "<VehLongComp_A_Actl>"

== system P702_NI_SoftECU/Output/Subsystem1/CAN_Signal/ABS_ESC/BrakeSnData_4_0x7D ==
  in_port : Inport
  BrkTotTqRqArb_No_Cnt : Terminator
  BrkTotTqRqArb_No_Cs : Terminator
  BrkTot_Tq_Actl : Terminator
  BrkTot_Tq_RqArb : Terminator
  HsaStat_D_Actl : Terminator
  VehRolComp_W_Actl : Terminator
  VehVertComp_A_Actl : Terminator
  bus_selector : BusSelector  OutputSignals=HsaStat_D_Actl,BrkTot_Tq_RqArb,BrkTotTqRqArb_No_Cs,BrkTotTqRqArb_No_Cnt,BrkTot_Tq_Actl,VehVertComp_A_Actl,VehRolComp_W_Actl
  wires:
  in_port/1 -> bus_selector/1  "Subsystem1"
  bus_selector/1 -> HsaStat_D_Actl/1  "<HsaStat_D_Actl>"
  bus_selector/2 -> BrkTot_Tq_RqArb/1  "<BrkTot_Tq_RqArb>"
  bus_selector/3 -> BrkTotTqRqArb_No_Cs/1  "<BrkTotTqRqArb_No_Cs>"
  bus_selector/4 -> BrkTotTqRqArb_No_Cnt/1  "<BrkTotTqRqArb_No_Cnt>"
  bus_selector/5 -> BrkTot_Tq_Actl/1  "<BrkTot_Tq_Actl>"
  bus_selector/6 -> VehVertComp_A_Actl/1  "<VehVertComp_A_Actl>"
  bus_selector/7 -> VehRolComp_W_Actl/1  "<VehRolComp_W_Actl>"

== system P702_NI_SoftECU/Output/Subsystem1/CAN_Signal/ABS_ESC/BrakeSnData_5_0x76 ==
  in_port : Inport
  AwdLck_Tq_RqMn : Terminator
  AwdLck_Tq_RqMx : Terminator
  BrkCtrFnd_B_Stat : Terminator
  DrvSte_D_Stat : Terminator
  DrvSte_Tq_Rq : Terminator
  EmgcyBrkLamp_D_Rq : Terminator
  SteWhlCompAnEst_D_Qf : Terminator
  SteWhlComp_An_Est : Terminator
  StopLamp_B_RqBrk : Terminator
  bus_selector : BusSelector  OutputSignals=StopLamp_B_RqBrk,SteWhlComp_An_Est,SteWhlCompAnEst_D_Qf,EmgcyBrkLamp_D_Rq,DrvSte_D_Stat,DrvSte_Tq_Rq,BrkCtrFnd_B_Stat,AwdLck_Tq_RqMx,AwdLck_Tq_RqMn
  wires:
  in_port/1 -> bus_selector/1  "Subsystem1"
  bus_selector/1 -> StopLamp_B_RqBrk/1  "<StopLamp_B_RqBrk>"
  bus_selector/2 -> SteWhlComp_An_Est/1  "<SteWhlComp_An_Est>"
  bus_selector/3 -> SteWhlCompAnEst_D_Qf/1  "<SteWhlCompAnEst_D_Qf>"
  bus_selector/4 -> EmgcyBrkLamp_D_Rq/1  "<EmgcyBrkLamp_D_Rq>"
  bus_selector/5 -> DrvSte_D_Stat/1  "<DrvSte_D_Stat>"
  bus_selector/6 -> DrvSte_Tq_Rq/1  "<DrvSte_Tq_Rq>"
  bus_selector/7 -> BrkCtrFnd_B_Stat/1  "<BrkCtrFnd_B_Stat>"
  bus_selector/8 -> AwdLck_Tq_RqMx/1  "<AwdLck_Tq_RqMx>"
  bus_selector/9 -> AwdLck_Tq_RqMn/1  "<AwdLck_Tq_RqMn>"

== system P702_NI_SoftECU/Output/Subsystem1/CAN_Signal/ABS_ESC/BrakeSnData_6_0x414 ==
  in_port : Inport
  StePinOffst_An_Est : Terminator
  StePinOffst_D_Stat : Terminator
  StePinOffst_No_Cnt : Terminator
  StePinOffst_No_Cs : Terminator
  bus_selector : BusSelector  OutputSignals=StePinOffst_An_Est,StePinOffst_D_Stat,StePinOffst_No_Cnt,StePinOffst_No_Cs
  wires:
  in_port/1 -> bus_selector/1  "Subsystem1"
  bus_selector/1 -> StePinOffst_An_Est/1  "<StePinOffst_An_Est>"
  bus_selector/2 -> StePinOffst_D_Stat/1  "<StePinOffst_D_Stat>"
  bus_selector/3 -> StePinOffst_No_Cnt/1  "<StePinOffst_No_Cnt>"
  bus_selector/4 -> StePinOffst_No_Cs/1  "<StePinOffst_No_Cs>"

== system P702_NI_SoftECU/Output/Subsystem1/CAN_Signal/ABS_ESC/BrakeSysFeatures_0x415 ==
  in_port : Inport
  BrkFluidLvl_D_Stat : Terminator
  LsmcBrkDecel_D_Stat : Terminator
  VehStab_D_Stat : Terminator
  VehVActlBrk_D_Qf : Terminator
  VehVActlBrk_No_Cnt : Terminator
  VehVActlBrk_No_Cs : Terminator
  VehYawLin_W_Rq : Terminator
  VehYawNonLin_W_Rq : Terminator
  Veh_V_ActlBrk : Terminator
  bus_selector : BusSelector  OutputSignals=Veh_V_ActlBrk,VehVActlBrk_D_Qf,VehVActlBrk_No_Cnt,BrkFluidLvl_D_Stat,VehVActlBrk_No_Cs,LsmcBrkDecel_D_Stat,VehYawLin_W_Rq,VehStab_D_Stat,VehYawNonLin_W_Rq
  wires:
  in_port/1 -> bus_selector/1  "Subsystem1"
  bus_selector/1 -> Veh_V_ActlBrk/1  "<Veh_V_ActlBrk>"
  bus_selector/2 -> VehVActlBrk_D_Qf/1  "<VehVActlBrk_D_Qf>"
  bus_selector/3 -> VehVActlBrk_No_Cnt/1  "<VehVActlBrk_No_Cnt>"
  bus_selector/4 -> BrkFluidLvl_D_Stat/1  "<BrkFluidLvl_D_Stat>"
  bus_selector/5 -> VehVActlBrk_No_Cs/1  "<VehVActlBrk_No_Cs>"
  bus_selector/6 -> LsmcBrkDecel_D_Stat/1  "<LsmcBrkDecel_D_Stat>"
  bus_selector/7 -> VehYawLin_W_Rq/1  "<VehYawLin_W_Rq>"
  bus_selector/8 -> VehStab_D_Stat/1  "<VehStab_D_Stat>"
  bus_selector/9 -> VehYawNonLin_W_Rq/1  "<VehYawNonLin_W_Rq>"

== system P702_NI_SoftECU/Output/Subsystem1/CAN_Signal/ABS_ESC/BrakeSysFeatures_2_0x416 ==
  in_port : Inport
  Abs_B_Falt : Terminator
  BpedMove_D_Actl : Terminator
  BpedMove_No_Cnt : Terminator
  BrkBstrVac_B_Rq : Terminator
  BrkLamp_B_Rq : Terminator
  ChimeBrk_B_Rq : Terminator
  DrvAntiLckLamp_D_Rq : Terminator
  DrvHdcLampInfo_D_Rq : Terminator
  DrvHdcMsg_D_Rq : Terminator
  DrvHdcWarnInfo_D_Rq : Terminator
  DrvSlipCtlLamp_D_Rq : Terminator
  DrvSlipCtlMde_D_Ind : Terminator
  HILL_DESC_MC : Terminator
  HdcMde_D_Actl : Terminator
  HsaMde_D_Mem : Terminator
  RearDiffElckrOpen_B_Rq : Terminator
  RearDiffLck_Tq2_RqMx : Terminator
  StabCtlBrk_B_Avail : Terminator
  TCMode : Terminator
  TRLR_SWAY_CONFIG_STAT : Terminator
  TRLR_SWAY_EVNT_IN_PROG : Terminator
  bus_selector : BusSelector  OutputSignals=BpedMove_D_Actl,Abs_B_Falt,StabCtlBrk_B_Avail,BpedMove_No_Cnt,TCMode,ChimeBrk_B_Rq,BrkLamp_B_Rq,DrvHdcLampInfo_D_Rq,DrvHdcMsg_D_Rq,HdcMde_D_Actl,BrkBstrVac_B_Rq,TRLR_SWAY_CONFIG_STAT,TRLR_SWAY_EVNT_IN_PROG,DrvHdcWarnInfo_D_Rq,HsaMde_D_Mem,HILL_DESC_MC,DrvSlipCtlMde_D_Ind,DrvSlipCtlLamp_D_Rq,RearDiffElckrOpen_B_Rq,DrvAntiLckLamp_D_Rq,RearDiffLck_Tq2_RqMx
  wires:
  in_port/1 -> bus_selector/1  "Subsystem1"
  bus_selector/1 -> BpedMove_D_Actl/1  "<BpedMove_D_Actl>"
  bus_selector/2 -> Abs_B_Falt/1  "<Abs_B_Falt>"
  bus_selector/3 -> StabCtlBrk_B_Avail/1  "<StabCtlBrk_B_Avail>"
  bus_selector/4 -> BpedMove_No_Cnt/1  "<BpedMove_No_Cnt>"
  bus_selector/5 -> TCMode/1  "<TCMode>"
  bus_selector/6 -> ChimeBrk_B_Rq/1  "<ChimeBrk_B_Rq>"
  bus_selector/7 -> BrkLamp_B_Rq/1  "<BrkLamp_B_Rq>"
  bus_selector/8 -> DrvHdcLampInfo_D_Rq/1  "<DrvHdcLampInfo_D_Rq>"
  bus_selector/9 -> DrvHdcMsg_D_Rq/1  "<DrvHdcMsg_D_Rq>"
  bus_selector/10 -> HdcMde_D_Actl/1  "<HdcMde_D_Actl>"
  bus_selector/11 -> BrkBstrVac_B_Rq/1  "<BrkBstrVac_B_Rq>"
  bus_selector/12 -> TRLR_SWAY_CONFIG_STAT/1  "<TRLR_SWAY_CONFIG_STAT>"
  bus_selector/13 -> TRLR_SWAY_EVNT_IN_PROG/1  "<TRLR_SWAY_EVNT_IN_PROG>"
  bus_selector/14 -> DrvHdcWarnInfo_D_Rq/1  "<DrvHdcWarnInfo_D_Rq>"
  bus_selector/15 -> HsaMde_D_Mem/1  "<HsaMde_D_Mem>"
  bus_selector/16 -> HILL_DESC_MC/1  "<HILL_DESC_MC>"
  bus_selector/17 -> DrvSlipCtlMde_D_Ind/1  "<DrvSlipCtlMde_D_Ind>"
  bus_selector/18 -> DrvSlipCtlLamp_D_Rq/1  "<DrvSlipCtlLamp_D_Rq>"
  bus_selector/19 -> RearDiffElckrOpen_B_Rq/1  "<RearDiffElckrOpen_B_Rq>"
  bus_selector/20 -> DrvAntiLckLamp_D_Rq/1  "<DrvAntiLckLamp_D_Rq>"
  bus_selector/21 -> RearDiffLck_Tq2_RqMx/1  "<RearDiffLck_Tq2_RqMx>"

== system P702_NI_SoftECU/Output/Subsystem1/CAN_Signal/ABS_ESC/BrakeSysFeatures_3_0x41E ==
  in_port : Inport
  ApaBrk_D_Stat : Terminator
  AutoHoldMde_D_Ind : Terminator
  AutoHoldMsgTxt_D_Rq : Terminator
  AutoHoldSwMde_B_Ind : Terminator
  BrkBstrVac_D_Stat : Terminator
  BrkMdeInhbt_B_RqDsply : Terminator
  CtaBrk_D_Stat : Terminator
  DrvSlipCtlMdeMsg_D_Rq : Terminator
  DrvSlipCtlOffLamp_D_Rq : Terminator
  RbaBrk_D_Stat : Terminator
  SelDrvMdeAwd_D_Rq : Terminator
  SelDrvMdeChassis2_D_Rq : Terminator
  SelDrvMdeChassis_D_Rq : Terminator
  TrailCtlMsgTxt_D_Rq : Terminator
  TrailCtl_D_Stat : Terminator
  bus_selector : BusSelector  OutputSignals=AutoHoldMsgTxt_D_Rq,AutoHoldSwMde_B_Ind,AutoHoldMde_D_Ind,DrvSlipCtlMdeMsg_D_Rq,BrkMdeInhbt_B_RqDsply,DrvSlipCtlOffLamp_D_Rq,BrkBstrVac_D_Stat,SelDrvMdeAwd_D_Rq,SelDrvMdeChassis_D_Rq,ApaBrk_D_Stat,CtaBrk_D_Stat,SelDrvMdeChassis2_D_Rq,TrailCtl_D_Stat,TrailCtlMsgTxt_D_Rq,RbaBrk_D_Stat
  wires:
  in_port/1 -> bus_selector/1  "Subsystem1"
  bus_selector/1 -> AutoHoldMsgTxt_D_Rq/1  "<AutoHoldMsgTxt_D_Rq>"
  bus_selector/2 -> AutoHoldSwMde_B_Ind/1  "<AutoHoldSwMde_B_Ind>"
  bus_selector/3 -> AutoHoldMde_D_Ind/1  "<AutoHoldMde_D_Ind>"
  bus_selector/4 -> DrvSlipCtlMdeMsg_D_Rq/1  "<DrvSlipCtlMdeMsg_D_Rq>"
  bus_selector/5 -> BrkMdeInhbt_B_RqDsply/1  "<BrkMdeInhbt_B_RqDsply>"
  bus_selector/6 -> DrvSlipCtlOffLamp_D_Rq/1  "<DrvSlipCtlOffLamp_D_Rq>"
  bus_selector/7 -> BrkBstrVac_D_Stat/1  "<BrkBstrVac_D_Stat>"
  bus_selector/8 -> SelDrvMdeAwd_D_Rq/1  "<SelDrvMdeAwd_D_Rq>"
  bus_selector/9 -> SelDrvMdeChassis_D_Rq/1  "<SelDrvMdeChassis_D_Rq>"
  bus_selector/10 -> ApaBrk_D_Stat/1  "<ApaBrk_D_Stat>"
  bus_selector/11 -> CtaBrk_D_Stat/1  "<CtaBrk_D_Stat>"
  bus_selector/12 -> SelDrvMdeChassis2_D_Rq/1  "<SelDrvMdeChassis2_D_Rq>"
  bus_selector/13 -> TrailCtl_D_Stat/1  "<TrailCtl_D_Stat>"
  bus_selector/14 -> TrailCtlMsgTxt_D_Rq/1  "<TrailCtlMsgTxt_D_Rq>"
  bus_selector/15 -> RbaBrk_D_Stat/1  "<RbaBrk_D_Stat>"

== system P702_NI_SoftECU/Output/Subsystem1/CAN_Signal/ABS_ESC/DesiredTorqBrk_0x213 ==
  in_port : Inport
  AbsActv_B_Actl : Terminator
  AccBrkActv_B_Actl : Terminator
  AccBrkDeny_B_Actl : Terminator
  AccBrkDis_B_Actl : Terminator
  AccBrkPrchgActv_B_Actl : Terminator
  AccBrkTotTqMn_B_Actl : Terminator
  AccBrkWarm_B_Actl : Terminator
  AccDis_B_ActlEpb : Terminator
  AccStopActv_B_ActlBrk : Terminator
  CcDis_B_Cmd : Terminator
  CmbbBaSensInc_B_Actl : Terminator
  CmbbBrkDecel_B_Actl : Terminator
  CmbbBrkDis_B_Actl : Terminator
  CmbbBrkPrchg_B_Actl : Terminator
  CmbbDeny_B_ActlBrk : Terminator
  LscmbBrkPrchg_B_Actl : Terminator
  LscmbbBaSensInc_B_Actl : Terminator
  LscmbbBrkDecel_B_Actl : Terminator
  LscmbbBrkDis_B_Actl : Terminator
  LscmbbDeny_B_ActlBrk : Terminator
  LscmbbMntr_B_Err : Terminator
  PrkBrkMsgTxt_D_Rq : Terminator
  PrkBrkRedLamp_D_Rq : Terminator
  PrkBrkStatus : Terminator
  PrkBrkYwLamp_D_Rq : Terminator
  PrplDrgCtlActv_B_Actl : Terminator
  PrplWhlTot_Tq_RqMx : Terminator
  StabCtlBrkActv_B_Actl : Terminator
  TracCtlPtActv_B_Actl : Terminator
  VehLongOvrGnd_A_Est : Terminator
  VehStop_D_Stat : Terminator
  VehicleStationary : Terminator
  bus_selector : BusSelector  OutputSignals=PrplWhlTot_Tq_RqMx,StabCtlBrkActv_B_Actl,AccStopActv_B_ActlBrk,LscmbbBaSensInc_B_Actl,LscmbbBrkDecel_B_Actl,LscmbbBrkDis_B_Actl,LscmbbDeny_B_ActlBrk,LscmbbMntr_B_Err,LscmbBrkPrchg_B_Actl,TracCtlPtActv_B_Actl,PrkBrkRedLamp_D_Rq,VehStop_D_Stat,PrkBrkStatus,VehicleStationary,PrkBrkYwLamp_D_Rq,PrkBrkMsgTxt_D_Rq,AccDis_B_ActlEpb,CcDis_B_Cmd,PrplDrgCtlActv_B_Actl,AbsActv_B_Actl,AccBrkDis_B_Actl,AccBrkActv_B_Actl,AccBrkDeny_B_Actl,VehLongOvrGnd_A_Est,AccBrkWarm_B_Actl,AccBrkTotTqMn_B_Actl,AccBrkPrchgActv_B_Actl,CmbbDeny_B_ActlBrk,CmbbBrkPrchg_B_Actl,CmbbBrkDecel_B_Actl,CmbbBaSensInc_B_Actl,CmbbBrkDis_B_Actl
  wires:
  in_port/1 -> bus_selector/1  "Subsystem1"
  bus_selector/1 -> PrplWhlTot_Tq_RqMx/1  "<PrplWhlTot_Tq_RqMx>"
  bus_selector/2 -> StabCtlBrkActv_B_Actl/1  "<StabCtlBrkActv_B_Actl>"
  bus_selector/3 -> AccStopActv_B_ActlBrk/1  "<AccStopActv_B_ActlBrk>"
  bus_selector/4 -> LscmbbBaSensInc_B_Actl/1  "<LscmbbBaSensInc_B_Actl>"
  bus_selector/5 -> LscmbbBrkDecel_B_Actl/1  "<LscmbbBrkDecel_B_Actl>"
  bus_selector/6 -> LscmbbBrkDis_B_Actl/1  "<LscmbbBrkDis_B_Actl>"
  bus_selector/7 -> LscmbbDeny_B_ActlBrk/1  "<LscmbbDeny_B_ActlBrk>"
  bus_selector/8 -> LscmbbMntr_B_Err/1  "<LscmbbMntr_B_Err>"
  bus_selector/9 -> LscmbBrkPrchg_B_Actl/1  "<LscmbBrkPrchg_B_Actl>"
  bus_selector/10 -> TracCtlPtActv_B_Actl/1  "<TracCtlPtActv_B_Actl>"
  bus_selector/11 -> PrkBrkRedLamp_D_Rq/1  "<PrkBrkRedLamp_D_Rq>"
  bus_selector/12 -> VehStop_D_Stat/1  "<VehStop_D_Stat>"
  bus_selector/13 -> PrkBrkStatus/1  "<PrkBrkStatus>"
  bus_selector/14 -> VehicleStationary/1  "<VehicleStationary>"
  bus_selector/15 -> PrkBrkYwLamp_D_Rq/1  "<PrkBrkYwLamp_D_Rq>"
  bus_selector/16 -> PrkBrkMsgTxt_D_Rq/1  "<PrkBrkMsgTxt_D_Rq>"
  bus_selector/17 -> AccDis_B_ActlEpb/1  "<AccDis_B_ActlEpb>"
  bus_selector/18 -> CcDis_B_Cmd/1  "<CcDis_B_Cmd>"
  bus_selector/19 -> PrplDrgCtlActv_B_Actl/1  "<PrplDrgCtlActv_B_Actl>"
  bus_selector/20 -> AbsActv_B_Actl/1  "<AbsActv_B_Actl>"
  bus_selector/21 -> AccBrkDis_B_Actl/1  "<AccBrkDis_B_Actl>"
  bus_selector/22 -> AccBrkActv_B_Actl/1  "<AccBrkActv_B_Actl>"
  bus_selector/23 -> AccBrkDeny_B_Actl/1  "<AccBrkDeny_B_Actl>"
  bus_selector/24 -> VehLongOvrGnd_A_Est/1  "<VehLongOvrGnd_A_Est>"
  bus_selector/25 -> AccBrkWarm_B_Actl/1  "<AccBrkWarm_B_Actl>"
  bus_selector/26 -> AccBrkTotTqMn_B_Actl/1  "<AccBrkTotTqMn_B_Actl>"
  bus_selector/27 -> AccBrkPrchgActv_B_Actl/1  "<AccBrkPrchgActv_B_Actl>"
  bus_selector/28 -> CmbbDeny_B_ActlBrk/1  "<CmbbDeny_B_ActlBrk>"
  bus_selector/29 -> CmbbBrkPrchg_B_Actl/1  "<CmbbBrkPrchg_B_Actl>"
  bus_selector/30 -> CmbbBrkDecel_B_Actl/1  "<CmbbBrkDecel_B_Actl>"
  bus_selector/31 -> CmbbBaSensInc_B_Actl/1  "<CmbbBaSensInc_B_Actl>"
  bus_selector/32 -> CmbbBrkDis_B_Actl/1  "<CmbbBrkDis_B_Actl>"

== system P702_NI_SoftECU/Output/Subsystem1/CAN_Signal/ABS_ESC/DesiredTorqBrk_2_0x214 ==
  in_port : Inport
  PrplWhlRear_Tq_RqMn : Terminator
  PrplWhlRear_Tq_RqMx : Terminator
  PrplWhlTot_Tq_RqMn : Terminator
  PrplWhlTqRqMn_No_Cnt : Terminator
  PrplWhlTqRqMn_No_Cs : Terminator
  RgenBrkDynoMde_B_Actl : Terminator
  RgenTqFalt_B_Actl : Terminator
  bus_selector : BusSelector  OutputSignals=PrplWhlTot_Tq_RqMn,PrplWhlRear_Tq_RqMx,PrplWhlRear_Tq_RqMn,PrplWhlTqRqMn_No_Cs,PrplWhlTqRqMn_No_Cnt,RgenTqFalt_B_Actl,RgenBrkDynoMde_B_Actl
  wires:
  in_port/1 -> bus_selector/1  "Subsystem1"
  bus_selector/1 -> PrplWhlTot_Tq_RqMn/1  "<PrplWhlTot_Tq_RqMn>"
  bus_selector/2 -> PrplWhlRear_Tq_RqMx/1  "<PrplWhlRear_Tq_RqMx>"
  bus_selector/3 -> PrplWhlRear_Tq_RqMn/1  "<PrplWhlRear_Tq_RqMn>"
  bus_selector/4 -> PrplWhlTqRqMn_No_Cs/1  "<PrplWhlTqRqMn_No_Cs>"
  bus_selector/5 -> PrplWhlTqRqMn_No_Cnt/1  "<PrplWhlTqRqMn_No_Cnt>"
  bus_selector/6 -> RgenTqFalt_B_Actl/1  "<RgenTqFalt_B_Actl>"
  bus_selector/7 -> RgenBrkDynoMde_B_Actl/1  "<RgenBrkDynoMde_B_Actl>"
